simulink model "actividad_2"  (R2012b)
settings: Solver=ode45  StartTime=0.0  StopTime=10.0  RelTol=1e-3
libraries: simulink x2, vipviewers_win32 x1
settings Model: Creator=usuario  LastModifiedBy=usuario

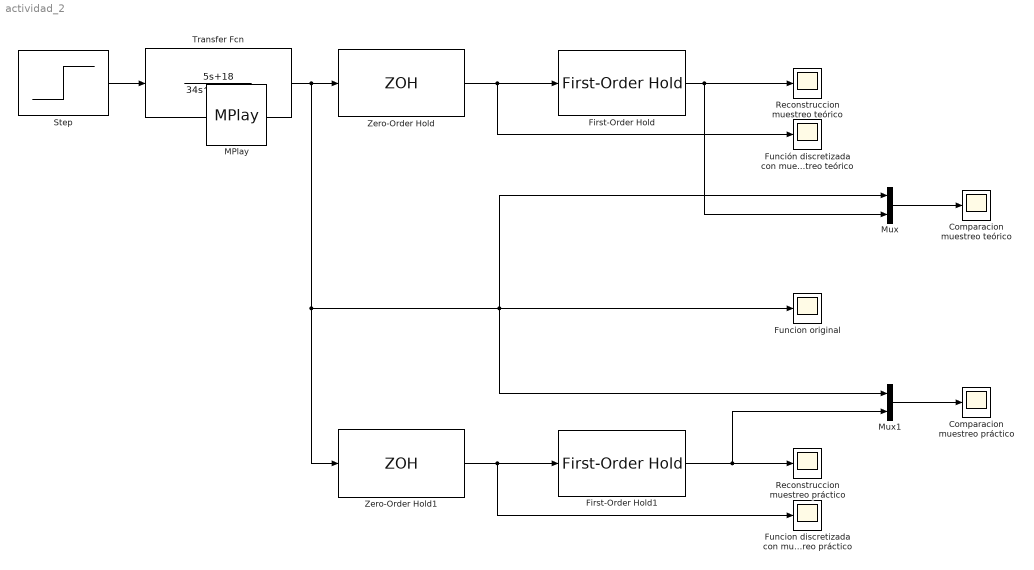
== system actividad_2 ==
  Comparacion muestreo práctico : Scope
      settings: ShowLegends=on  SaveName=ScopeData6
  Comparacion muestreo teórico : Scope
      settings: ShowLegends=on  SaveName=ScopeData7
  First-Order Hold : simulink/Discrete/First-Order Hold  DisableCoverage=on  Ts=3.685
  First-Order Hold1 : simulink/Discrete/First-Order Hold  DisableCoverage=on  Ts=0.3685
  Funcion discretizada con muestreo práctico : Scope
      settings: SaveName=ScopeData4
  "Funcion original " : Scope
      settings: SaveName=ScopeData2
  Función discretizada con muestreo teórico : Scope
  Mux : Mux  Inputs=2
  Mux1 : Mux  Inputs=2
  Reconstruccion muestreo práctico : Scope
      settings: SaveName=ScopeData3
  "Reconstruccion muestreo teórico " : Scope
  Step : Step  SampleTime=0
  Transfer Fcn : TransferFcn  Numerator=[5 18]  Denominator=[34 -6 25]
  Zero-Order Hold : ZeroOrderHold  SampleTime=3.685
  Zero-Order Hold1 : ZeroOrderHold  SampleTime=0.3685
  MPlay : vipviewers_win32/MPlay  IOType=viewer  ShowInLibBrowser=off
  wires:
  Step/1 -> Transfer Fcn/1
  First-Order Hold/1 -> Mux/2, "Reconstruccion muestreo teórico "/1
  Zero-Order Hold/1 -> Función discretizada con muestreo teórico/1, First-Order Hold/1
  First-Order Hold1/1 -> Mux1/2, Reconstruccion muestreo práctico/1
  Zero-Order Hold1/1 -> Funcion discretizada con muestreo práctico/1, First-Order Hold1/1
  Transfer Fcn/1 -> Zero-Order Hold1/1, Mux1/1, Mux/1, "Funcion original "/1, Zero-Order Hold/1
  Mux/1 -> Comparacion muestreo teórico/1
  Mux1/1 -> Comparacion muestreo práctico/1
